simulink library "FuelSystemLibrary"  (R2014b)
settings: Solver=ode45  SolverMode=SingleTasking  StartTime=0.0  StopTime=10.0  RelTol=1e-3
undefined symbols (not defined in the file): BooleanOff, BooleanOn, BoolThreshold, BowserOnPressure, CouplingOffPressure, CouplingOnPressure, DefaultTemp, DiffuserResistance, DiscreteSwitchOff, DiscreteSwitchOn, DiscreteSwitchThreshold, FloatingPressure, FlowNoOverride, FspSamplingPeriod, FuelSpecificHeatCapacity, g, InfiniteFlow, InfiniteMass, InfiniteResistance, InfiniteTime, InfiniteVolume, kpl2kpm3, MaxAValue, MaxBValue, MeterNoReset, MinAValue, MinBValue, NearZeroMass, NearZeroTime, NoError, NominalAValue, NominalBValue, NonRetResistance, NoReset, NullBasePress, PerCycle2PerSec, PerSec2PerCycle, PipeDisconnected, PipeResistance, PumpOnTime, TankFixedMassError, TankInletResistance, TankInstPortStartOffset, TankNoReset, TypicalFuelDensity, ValveClosedPosition, ValveOnResistance, ValveOpenPosition, ValveOpenTime
libraries: FuelSystemLibrary x251, WrightSolverLib x50, simulink x1
(part 4 of 4)

== system FuelSystemLibrary/TankCore/ResetOveride : Subsys ==
  Default : Inport
  Reset : Inport  Port=2
  Override : Inport  Port=3
  Constant10 : Constant  Value=TankNoReset
  Relational Operator2 : RelationalOperator  Operator===  InputSameDT=on
  Select any reset signal : MinMax  Function=max  Inputs=2  SaturateOnIntegerOverflow=on  InputSameDT=on
  Switch3 : Switch  Threshold=BoolThreshold  SaturateOnIntegerOverflow=on  InputSameDT=on
  Out : Outport
  wires:
  Switch3/1 -> Out/1
  Default/1 -> Switch3/1
  Relational Operator2/1 -> Switch3/2
  Constant10/1 -> Relational Operator2/1
  Reset/1 -> Select any reset signal/1
  Override/1 -> Select any reset signal/2
  Select any reset signal/1 -> Relational Operator2/2, Switch3/3

== system FuelSystemLibrary/Valve2Ip/ValveHead1 ==
  note: Enable valve conducting as soon as
      | the valve comes off the fully-closed position
  note: Valve head position->status calculation
  note: Slew direction calculation
  note: Valve position/conductance calculation
  note: Calculate flap position,
      | based on error condition
  note: Valve Error Decodes:
      | 0 - NoError
      | 1 - Flap Open
      | 2 - Flap Shut
  note: ValveHead - Calculation of Valve status and position
      |
      | Revision History -
      | Issue 1.0 - ?? - SW - Initial Issue
      | Issue1.1 - 28th October 2005 - DR - Added to FSP Generic Library
  En : Inport
  Flow : Inport  Port=2
  Closed Position : Constant  Value=ValveClosedPosition
  Const : Constant
  Const1 : Constant  Value=0
  Constant2 : Constant  Value=DiscreteSwitchOn
  Constant4 : Constant  Value=DiscreteSwitchOn
  Constant5 : Constant  Value=DiscreteSwitchOff
  Demux2 : Demux
  Logical Operator : Logic  Operator=NOT  AllPortsSameDT=off
  Multiport Switch : MultiPortSwitch  DataPortOrder=Zero-based contiguous  zeroidx=on  SaturateOnIntegerOverflow=on
  Prevent div-by-zero : Saturate  UpperLimit=InfiniteTime  LowerLimit=FspSamplingPeriod/10
  Product : Product  Inputs=**/  SaturateOnIntegerOverflow=on  OutDataTypeStr=Inherit: Same as first input
  Relational Operator1 : RelationalOperator  Operator===  ZeroCross=off
  Relational Operator2 : RelationalOperator  Operator===  ZeroCross=off
  Relational Operator3 : RelationalOperator  Operator===  ZeroCross=off
  Sum : Sum  Inputs=|+-  SaturateOnIntegerOverflow=on
  Terminator : Terminator
  Valve Head Position : Subsystem  TreatAsAtomicUnit=on
  Open : Outport
  Shut : Outport  Port=2
  Pos : Outport  Port=3
  Conducting : Outport  Port=4
  wires:
  Relational Operator2/1 -> [ValveOpen]
  Relational Operator1/1 -> [ValveClosed]
  Constant4/1 -> Relational Operator2/2
  Constant5/1 -> Relational Operator1/2
  Product/1 -> Valve Head Position/1(Inc)
  Sum/1 -> Product/1
  Constant2/1 -> Product/2
  Prevent div-by-zero/1 -> Product/3
  Demux2/2 -> Sum/2  "OffEn"
  Demux2/1 -> Sum/1  "OnEn"
  En/1 -> Demux2/1
  Demux2/3 -> Prevent div-by-zero/1  "SwitchTime"
  Relational Operator3/1 -> Logical Operator/1
  Logical Operator/1 -> Conducting/1
  Demux2/4 -> [ErrorCode]  "ErrorCode"
  Closed Position/1 -> Relational Operator3/2
  [HeadPos] -> Relational Operator1/1, Relational Operator2/1
  [FlapPos] -> Relational Operator3/1
  Valve Head Position/1(Pos) -> [HeadPos]
  [ErrorCode] -> Multiport Switch/1
  [HeadPos] -> Multiport Switch/2
  Const/1 -> Multiport Switch/3
  Const1/1 -> Multiport Switch/4
  Multiport Switch/1 -> [FlapPos]
  Flow/1 -> Terminator/1  "Flow"
  [ValveOpen] -> Open/1  "Open"
  [ValveClosed] -> Shut/1  "Closed"
  [FlapPos] -> Pos/1

== system FuelSystemLibrary/Valve2Ip/ValveHead1/Valve Head Position ==
  Inc : Inport
  PerSec2PerCycle : Gain  Gain=PerSec2PerCycle  OutDataTypeStr=Inherit: Same as input  ParamDataTypeStr=Inherit: Same as input
  Saturation : Saturate  UpperLimit=ValveOpenPosition  LowerLimit=ValveClosedPosition
  Sum : Sum  Inputs=|++  SaturateOnIntegerOverflow=on
  Unit Delay : UnitDelay  InitialCondition=DiscreteSwitchOff  SampleTime=-1
  Pos : Outport
  wires:
  PerSec2PerCycle/1 -> Sum/1
  Sum/1 -> Saturation/1
  Saturation/1 -> Unit Delay/1
  Unit Delay/1 -> Sum/2, Pos/1
  Inc/1 -> PerSec2PerCycle/1
